simulink library "atmosphere2"  (R2024b)
settings: Solver=VariableStepAuto  StartTime=0.0  StopTime=10.0  RelTol=1e-3
libraries: $bdroot x14
settings Model: Creator=user  LastModifiedBy=user

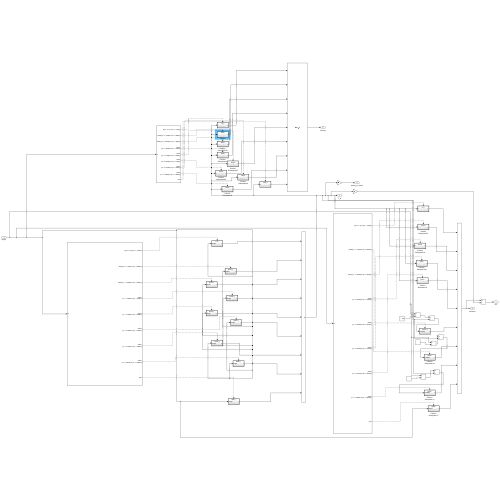
[thumbnail: Simulink's stored preview of the top-level diagram]
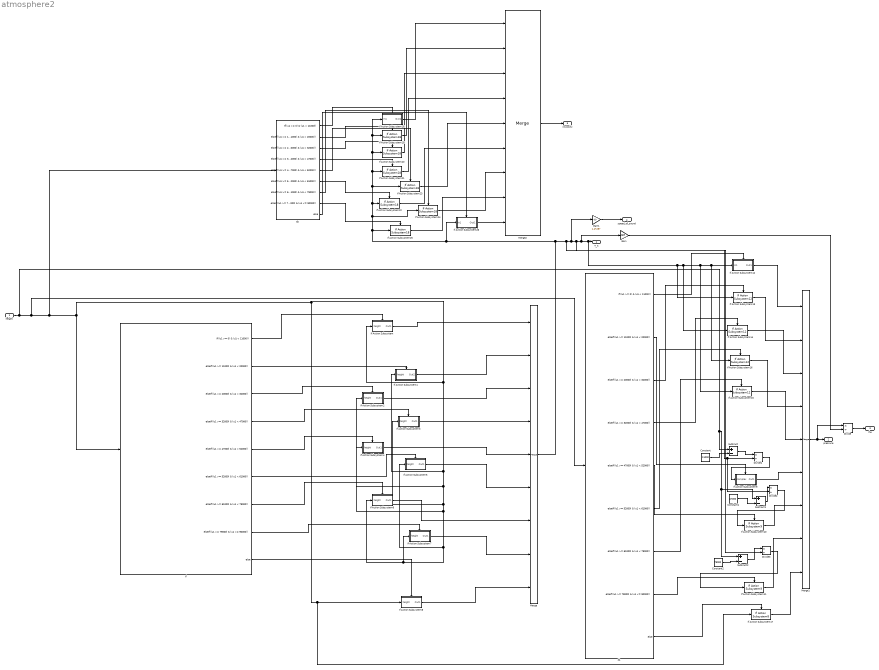
== system atmosphere2 ==
  height : Inport
  Constant : Constant  Value=11000
  Constant1 : Constant  Value=47000
  Constant2 : Constant  Value=79000
  Divide{,1..3} (4 alike) : Product  Inputs=*/
  Gain : Gain  Gain=287
  Gain1 : Gain  Gain=1.4*287
  If : If  IfExpression=(u1 >= 0) & (u1 < 11000)  ElseIfExpressions=|
      | (u1 >= 11000) & (u1 < 20000), (u1 >= 20000) & (u1 < 32000),
      | (u1 >= 32000) & (u1 < 47000),
      | (u1 >= 47000) & (u1 < 52000),
      | (u1 >= 52000) & (u1 < 61000),
      | (u1 >= 61000) & (u1 < 79000),
      | (u1 >= 79000) & (u1 <= 90000)
  If Action Subsystem : Subsystem  TreatAsAtomicUnit=on
  If Action Subsystem1 : Subsystem  TreatAsAtomicUnit=on
  If Action Subsystem10 : $bdroot/If Action Subsystem9  SystemSampleTime=-1  VariantActivationTime=update diagram  AllowFlexibleInterface=on  Latency=0  AutoFrameSizeCalculation=off
      link override Constant: Value=47000
      link override Gain: Gain=110.91
  If Action Subsystem11 : $bdroot/If Action Subsystem9  SystemSampleTime=-1  VariantActivationTime=update diagram  AllowFlexibleInterface=on  Latency=0  AutoFrameSizeCalculation=off
      link override Gain: Gain=0.373
  If Action Subsystem12 : Subsystem  TreatAsAtomicUnit=on
  If Action Subsystem13 : $bdroot/If Action Subsystem12  SystemSampleTime=-1  VariantActivationTime=update diagram  AllowFlexibleInterface=on  Latency=0  AutoFrameSizeCalculation=off
      link override Constant: Value=216.65
      link override g//8r*K): Value=-9.80665/(0.001*287)
  If Action Subsystem14 : $bdroot/If Action Subsystem12  SystemSampleTime=-1  VariantActivationTime=update diagram  AllowFlexibleInterface=on  Latency=0  AutoFrameSizeCalculation=off
      link override Constant: Value=228.65
      link override Gain: Gain=868.02
      link override g//8r*K): Value=-9.80665/(-0.0028*287)
  If Action Subsystem15 : $bdroot/If Action Subsystem12  SystemSampleTime=-1  VariantActivationTime=update diagram  AllowFlexibleInterface=on  Latency=0  AutoFrameSizeCalculation=off
      link override Constant: Value=252.65
      link override Gain: Gain=1.82
      link override g//8r*K): Value=-9.80665/(-0.004*287)
  If Action Subsystem16 : $bdroot/If Action Subsystem12  SystemSampleTime=-1  VariantActivationTime=update diagram  AllowFlexibleInterface=on  Latency=0  AutoFrameSizeCalculation=off
      link override Constant: Value=270.65
      link override Gain: Gain=59
      link override g//8r*K): Value=-9.80665/(-0.002*287)
  If Action Subsystem17 : $bdroot/If Action Subsystem8  SystemSampleTime=-1  VariantActivationTime=update diagram  AllowFlexibleInterface=on  Latency=0  AutoFrameSizeCalculation=off
  If Action Subsystem18 : Subsystem  TreatAsAtomicUnit=on
  If Action Subsystem19 : $bdroot/If Action Subsystem18  SystemSampleTime=-1  VariantActivationTime=update diagram  AllowFlexibleInterface=on  Latency=0  AutoFrameSizeCalculation=off
      link override Constant: Value=216.65
      link override Constant2: Value=216.65
  If Action Subsystem2 : Subsystem  TreatAsAtomicUnit=on
  If Action Subsystem20 : $bdroot/If Action Subsystem18  SystemSampleTime=-1  VariantActivationTime=update diagram  AllowFlexibleInterface=on  Latency=0  AutoFrameSizeCalculation=off
      link override Constant: Value=216.65
      link override Constant2: Value=216.65
  If Action Subsystem21 : $bdroot/If Action Subsystem18  SystemSampleTime=-1  VariantActivationTime=update diagram  AllowFlexibleInterface=on  Latency=0  AutoFrameSizeCalculation=off
      link override Constant: Value=228.65
      link override Constant2: Value=228.65
  If Action Subsystem22 : $bdroot/If Action Subsystem18  SystemSampleTime=-1  VariantActivationTime=update diagram  AllowFlexibleInterface=on  Latency=0  AutoFrameSizeCalculation=off
      link override Constant: Value=270.65
      link override Constant2: Value=270.65
  If Action Subsystem23 : $bdroot/If Action Subsystem18  SystemSampleTime=-1  VariantActivationTime=update diagram  AllowFlexibleInterface=on  Latency=0  AutoFrameSizeCalculation=off
      link override Constant: Value=270.65
      link override Constant2: Value=270.65
  If Action Subsystem24 : $bdroot/If Action Subsystem18  SystemSampleTime=-1  VariantActivationTime=update diagram  AllowFlexibleInterface=on  Latency=0  AutoFrameSizeCalculation=off
      link override Constant: Value=180.65
      link override Constant2: Value=180.65
  If Action Subsystem25 : $bdroot/If Action Subsystem18  SystemSampleTime=-1  VariantActivationTime=update diagram  AllowFlexibleInterface=on  Latency=0  AutoFrameSizeCalculation=off
      link override Constant: Value=180.65
      link override Constant2: Value=180.65
  If Action Subsystem26 : Subsystem  TreatAsAtomicUnit=on
  If Action Subsystem3 : Subsystem  TreatAsAtomicUnit=on
  If Action Subsystem4 : Subsystem  TreatAsAtomicUnit=on
  If Action Subsystem5 : Subsystem  TreatAsAtomicUnit=on
  If Action Subsystem6 : Subsystem  TreatAsAtomicUnit=on
  If Action Subsystem7 : Subsystem  TreatAsAtomicUnit=on
  If Action Subsystem8 : Subsystem  TreatAsAtomicUnit=on
  If Action Subsystem9 : Subsystem  TreatAsAtomicUnit=on
  If1 : If  IfExpression=(u1 >= 0) & (u1 < 11000)  ElseIfExpressions=|
      | (u1 >= 11000) & (u1 < 20000), (u1 >= 20000) & (u1 < 32000),
      | (u1 >= 32000) & (u1 < 47000),
      | (u1 >= 47000) & (u1 < 52000),
      | (u1 >= 52000) & (u1 < 61000),
      | (u1 >= 61000) & (u1 < 79000),
      | (u1 >= 79000) & (u1 <= 90000)
  If2 : If  IfExpression=(u1 >= 0) & (u1 < 11000)  ElseIfExpressions=|
      | (u1 >= 11000) & (u1 < 20000), (u1 >= 20000) & (u1 < 32000),
      | (u1 >= 32000) & (u1 < 47000),
      | (u1 >= 47000) & (u1 < 52000),
      | (u1 >= 52000) & (u1 < 61000),
      | (u1 >= 61000) & (u1 < 79000),
      | (u1 >= 79000) & (u1 <= 90000)
  Merge : Merge  Inputs=9
  Merge1 : Merge  Inputs=9
  Merge2 : Merge  Inputs=9
  Subtract : Sum  Inputs=+-
  Subtract1 : Sum  Inputs=+-
  Subtract2 : Sum  Inputs=+-
  T_K : Outport
  pressure : Outport  Port=2
  rho : Outport  Port=3
  spead_of_sound : Outport  Port=4
  viscosity : Outport  Port=5
  wires:
  If/1 -> If Action Subsystem/Action
  If/2 -> If Action Subsystem1/Action
  If/3 -> If Action Subsystem2/Action
  If/4 -> If Action Subsystem3/Action
  If/5 -> If Action Subsystem4/Action
  If/6 -> If Action Subsystem5/Action
  If/7 -> If Action Subsystem6/Action
  If/8 -> If Action Subsystem7/Action
  If/9 -> If Action Subsystem8/Action
  height/1 -> Subtract2/1, Subtract1/1, Subtract/1, If1/1, If2/1, If Action Subsystem4/1("height "), If Action Subsystem7/1("height "), If Action Subsystem6/1("height "), If Action Subsystem5/1("height "), If Action Subsystem3/1("height "), If Action Subsystem2/1("height "), If Action Subsystem1/1("height "), If Action Subsystem/1("height "), If Action Subsystem17/1, If Action Subsystem8/1("height "), If/1
  Merge/1 -> Divide3/2, Gain1/1, Divide2/2, Divide1/2, Gain/1, If Action Subsystem13/1, If Action Subsystem14/1, If Action Subsystem15/1, If Action Subsystem16/1, If Action Subsystem12/1(In1), T_K/1, If Action Subsystem24/1, If Action Subsystem22/1, If Action Subsystem23/1, If Action Subsystem21/1, If Action Subsystem20/1, If Action Subsystem19/1, If Action Subsystem18/1(In1), If Action Subsystem25/1, If Action Subsystem26/1(In1)
  If Action Subsystem/1(Out1) -> Merge/1
  If Action Subsystem1/1(Out2) -> Merge/2
  If Action Subsystem2/1(Out1) -> Merge/3
  If Action Subsystem3/1(Out1) -> Merge/4
  If Action Subsystem4/1(Out1) -> Merge/5
  If Action Subsystem5/1(Out1) -> Merge/6
  If Action Subsystem6/1(Out1) -> Merge/7
  If Action Subsystem7/1(Out1) -> Merge/8
  If Action Subsystem8/1(Out1) -> Merge/9
  If1/1 -> If Action Subsystem12/Action
  If1/3 -> If Action Subsystem13/Action
  If1/4 -> If Action Subsystem14/Action
  If1/6 -> If Action Subsystem16/Action
  If1/7 -> If Action Subsystem15/Action
  Constant/1 -> Subtract/2
  Subtract/1 -> Divide1/1
  Divide1/1 -> If Action Subsystem9/1(complex)
  If1/2 -> If Action Subsystem9/Action
  If1/5 -> If Action Subsystem10/Action
  Constant1/1 -> Subtract1/2
  Subtract1/1 -> Divide2/1
  Divide2/1 -> If Action Subsystem10/1
  If1/8 -> If Action Subsystem11/Action
  Constant2/1 -> Subtract2/2
  Subtract2/1 -> Divide3/1
  Divide3/1 -> If Action Subsystem11/1
  If Action Subsystem12/1(Out1) -> Merge1/1
  If Action Subsystem13/1 -> Merge1/2
  If Action Subsystem14/1 -> Merge1/3
  If Action Subsystem16/1 -> Merge1/4
  If Action Subsystem15/1 -> Merge1/5
  If Action Subsystem9/1(Out1) -> Merge1/6
  If Action Subsystem10/1 -> Merge1/7
  If Action Subsystem11/1 -> Merge1/8
  If Action Subsystem17/1 -> Merge1/9
  Merge1/1 -> Divide/1, pressure/1
  If1/9 -> If Action Subsystem17/Action
  Divide/1 -> rho/1
  Gain1/1 -> spead_of_sound/1
  If2/1 -> If Action Subsystem18/Action
  If2/2 -> If Action Subsystem19/Action
  If2/3 -> If Action Subsystem20/Action
  If2/4 -> If Action Subsystem21/Action
  If2/5 -> If Action Subsystem23/Action
  If2/6 -> If Action Subsystem22/Action
  If2/7 -> If Action Subsystem24/Action
  If2/8 -> If Action Subsystem25/Action
  If2/9 -> If Action Subsystem26/Action
  If Action Subsystem18/1(Out1) -> Merge2/1
  If Action Subsystem19/1 -> Merge2/2
  If Action Subsystem20/1 -> Merge2/3
  If Action Subsystem21/1 -> Merge2/4
  If Action Subsystem23/1 -> Merge2/5
  If Action Subsystem22/1 -> Merge2/6
  If Action Subsystem24/1 -> Merge2/7
  If Action Subsystem25/1 -> Merge2/8
  If Action Subsystem26/1(Out1) -> Merge2/9
  Merge2/1 -> viscosity/1
  Gain/1 -> Divide/2

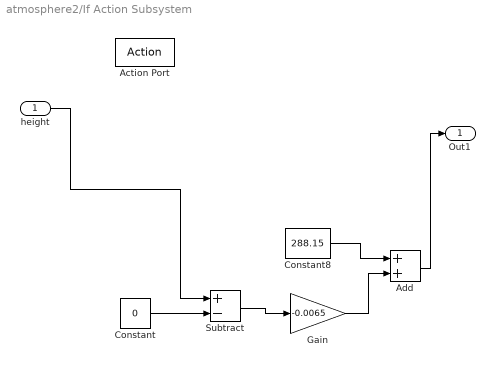
== system atmosphere2/If Action Subsystem ==
  "height " : Inport
  Action Port : ActionPort  ActionPortLabel=if((u1 >= 0) & (u1 < 11000))
  Add : Sum
  Constant : Constant  Value=0
  Constant8 : Constant  Value=288.15
  Gain : Gain  Gain=-0.0065
  Subtract : Sum  Inputs=+-
  Out1 : Outport
  wires:
  "height "/1 -> Subtract/1
  Constant/1 -> Subtract/2
  Subtract/1 -> Gain/1
  Gain/1 -> Add/2
  Constant8/1 -> Add/1
  Add/1 -> Out1/1

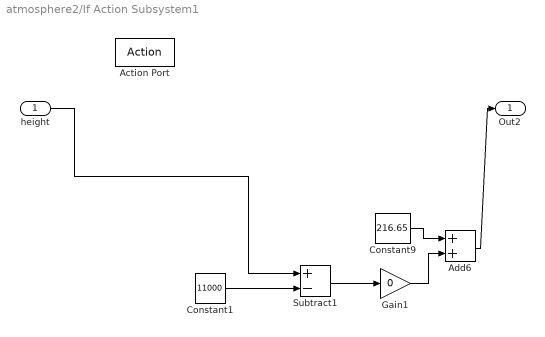
== system atmosphere2/If Action Subsystem1 ==
  "height " : Inport
  Action Port : ActionPort  ActionPortLabel=elseif((u1 >= 11000) & (u1 < 20000))
  Add6 : Sum
  Constant1 : Constant  Value=11000
  Constant9 : Constant  Value=216.65
  Gain1 : Gain  Gain=0
  Subtract1 : Sum  Inputs=+-
  Out2 : Outport
  wires:
  "height "/1 -> Subtract1/1
  Gain1/1 -> Add6/2
  Constant9/1 -> Add6/1
  Subtract1/1 -> Gain1/1
  Constant1/1 -> Subtract1/2
  Add6/1 -> Out2/1

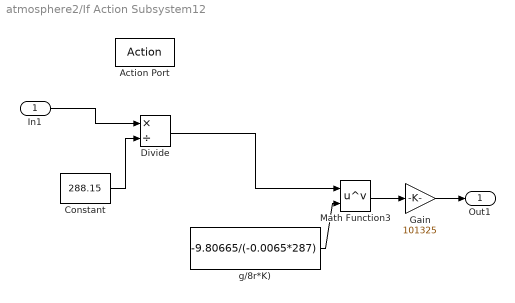
== system atmosphere2/If Action Subsystem12 ==
  In1 : Inport
  Action Port : ActionPort  ActionPortLabel=if((u1 >= 0) & (u1 < 11000))
  Constant : Constant  Value=288.15
  Divide : Product  Inputs=*/
  Gain : Gain  Gain=101325
  Math Function3 : Math  Operator=pow
  g/8r*K) : Constant  Value=-9.80665/(-0.0065*287)
  Out1 : Outport
  wires:
  In1/1 -> Divide/1
  Constant/1 -> Divide/2
  g/8r*K)/1 -> Math Function3/2
  Divide/1 -> Math Function3/1
  Math Function3/1 -> Gain/1
  Gain/1 -> Out1/1

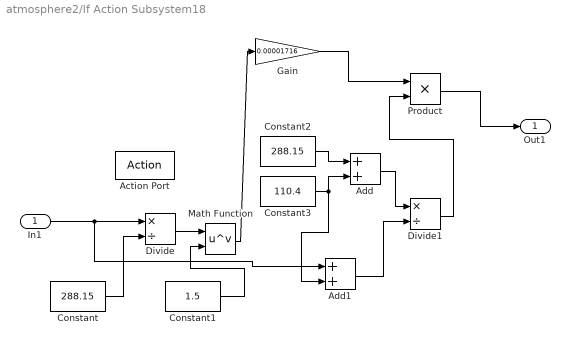
== system atmosphere2/If Action Subsystem18 ==
  In1 : Inport
  Action Port : ActionPort  ActionPortLabel=if((u1 >= 0) & (u1 < 11000))
  Add : Sum
  Add1 : Sum
  Constant : Constant  Value=288.15
  Constant1 : Constant  Value=1.5
  Constant2 : Constant  Value=288.15
  Constant3 : Constant  Value=110.4
  Divide : Product  Inputs=*/
  Divide1 : Product  Inputs=*/
  Gain : Gain  Gain=0.00001716
  Math Function : Math  Operator=pow
  Product : Product
  Out1 : Outport
  wires:
  In1/1 -> Add1/1, Divide/1
  Constant/1 -> Divide/2
  Divide/1 -> Math Function/1
  Constant1/1 -> Math Function/2
  Constant2/1 -> Add/1
  Constant3/1 -> Add/2, Add1/2
  Add/1 -> Divide1/1
  Add1/1 -> Divide1/2
  Divide1/1 -> Product/2
  Math Function/1 -> Gain/1
  Gain/1 -> Product/1
  Product/1 -> Out1/1

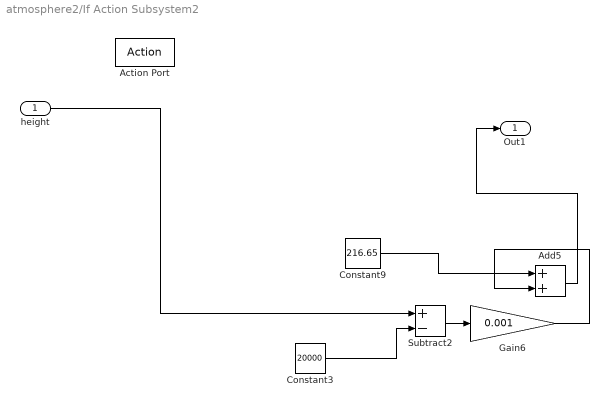
== system atmosphere2/If Action Subsystem2 ==
  "height " : Inport
  Action Port : ActionPort  ActionPortLabel=elseif( (u1 >= 20000) & (u1 < 32000))
  Add5 : Sum
  Constant3 : Constant  Value=20000
  Constant9 : Constant  Value=216.65
  Gain6 : Gain  Gain=0.001
  Subtract2 : Sum  Inputs=+-
  Out1 : Outport
  wires:
  Constant3/1 -> Subtract2/2
  Subtract2/1 -> Gain6/1
  Gain6/1 -> Add5/2
  Constant9/1 -> Add5/1
  "height "/1 -> Subtract2/1
  Add5/1 -> Out1/1

== system atmosphere2/If Action Subsystem26 ==
  In1 : Inport
  Action Port : ActionPort  ActionPortLabel=else
  Gain : Gain  Gain=0
  Out1 : Outport
  wires:
  In1/1 -> Gain/1
  Gain/1 -> Out1/1

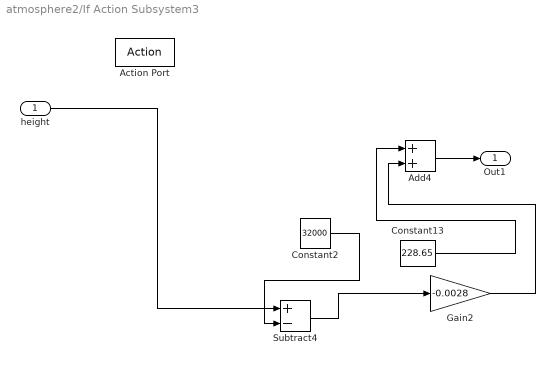
== system atmosphere2/If Action Subsystem3 ==
  "height " : Inport
  Action Port : ActionPort  ActionPortLabel=|
      | elseif(
      | (u1 >= 32000) & (u1 < 47000))
  Add4 : Sum
  Constant13 : Constant  Value=228.65
  Constant2 : Constant  Value=32000
  Gain2 : Gain  Gain=-0.0028
  Subtract4 : Sum  Inputs=+-
  Out1 : Outport
  wires:
  Subtract4/1 -> Gain2/1
  Constant2/1 -> Subtract4/2
  Constant13/1 -> Add4/1
  Gain2/1 -> Add4/2
  "height "/1 -> Subtract4/1
  Add4/1 -> Out1/1

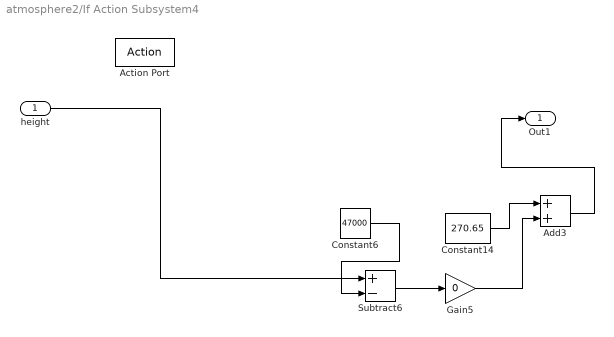
== system atmosphere2/If Action Subsystem4 ==
  "height " : Inport
  Action Port : ActionPort  ActionPortLabel=|
      | elseif(
      | (u1 >= 47000) & (u1 < 52000))
  Add3 : Sum
  Constant14 : Constant  Value=270.65
  Constant6 : Constant  Value=47000
  Gain5 : Gain  Gain=0
  Subtract6 : Sum  Inputs=+-
  Out1 : Outport
  wires:
  Subtract6/1 -> Gain5/1
  Constant14/1 -> Add3/1
  Constant6/1 -> Subtract6/2
  Gain5/1 -> Add3/2
  "height "/1 -> Subtract6/1
  Add3/1 -> Out1/1

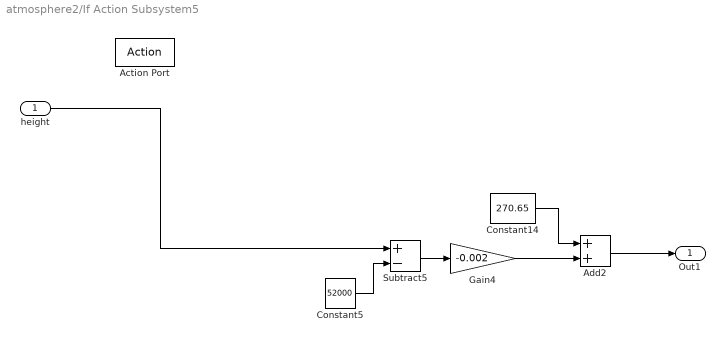
== system atmosphere2/If Action Subsystem5 ==
  "height " : Inport
  Action Port : ActionPort  ActionPortLabel=|
      | elseif(
      | (u1 >= 52000) & (u1 < 61000))
  Add2 : Sum
  Constant14 : Constant  Value=270.65
  Constant5 : Constant  Value=52000
  Gain4 : Gain  Gain=-0.002
  Subtract5 : Sum  Inputs=+-
  Out1 : Outport
  wires:
  Subtract5/1 -> Gain4/1
  Gain4/1 -> Add2/2
  Constant5/1 -> Subtract5/2
  Constant14/1 -> Add2/1
  "height "/1 -> Subtract5/1
  Add2/1 -> Out1/1

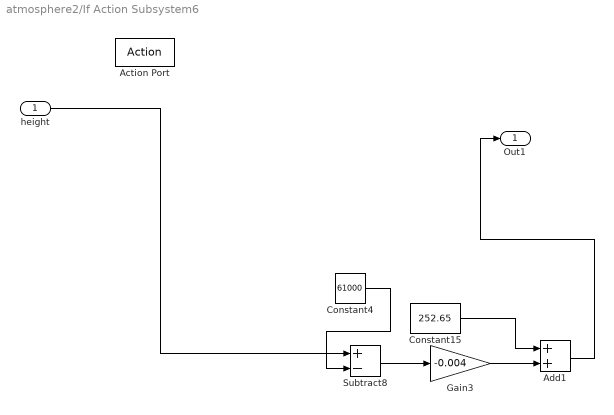
== system atmosphere2/If Action Subsystem6 ==
  "height " : Inport
  Action Port : ActionPort  ActionPortLabel=|
      | elseif(
      | (u1 >= 61000) & (u1 < 79000))
  Add1 : Sum
  Constant15 : Constant  Value=252.65
  Constant4 : Constant  Value=61000
  Gain3 : Gain  Gain=-0.004
  Subtract8 : Sum  Inputs=+-
  Out1 : Outport
  wires:
  Constant4/1 -> Subtract8/2
  Subtract8/1 -> Gain3/1
  Gain3/1 -> Add1/2
  Constant15/1 -> Add1/1
  "height "/1 -> Subtract8/1
  Add1/1 -> Out1/1

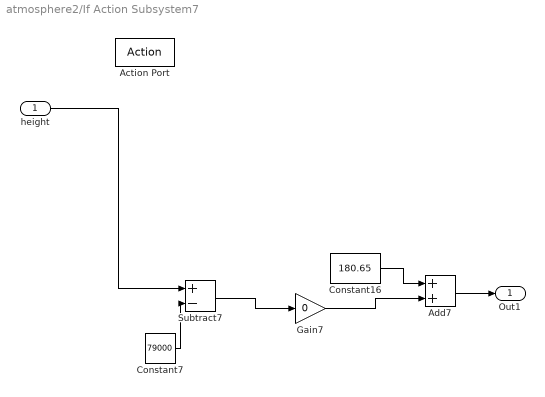
== system atmosphere2/If Action Subsystem7 ==
  "height " : Inport
  Action Port : ActionPort  ActionPortLabel=|
      | elseif(
      | (u1 >= 79000) & (u1 <= 90000))
  Add7 : Sum
  Constant16 : Constant  Value=180.65
  Constant7 : Constant  Value=79000
  Gain7 : Gain  Gain=0
  Subtract7 : Sum  Inputs=+-
  Out1 : Outport
  wires:
  Subtract7/1 -> Gain7/1
  Constant7/1 -> Subtract7/2
  Gain7/1 -> Add7/2
  Constant16/1 -> Add7/1
  "height "/1 -> Subtract7/1
  Add7/1 -> Out1/1

== system atmosphere2/If Action Subsystem8 ==
  "height " : Inport
  Action Port : ActionPort  ActionPortLabel=else
  Gain : Gain  Gain=0
  Out1 : Outport
  wires:
  "height "/1 -> Gain/1
  Gain/1 -> Out1/1

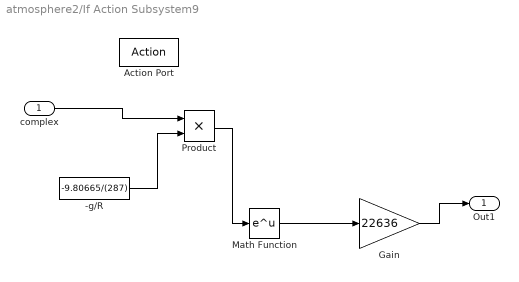
== system atmosphere2/If Action Subsystem9 ==
  complex : Inport
  Action Port : ActionPort  ActionPortLabel=elseif((u1 >= 11000) & (u1 < 20000))
  -g/R : Constant  Value=-9.80665/(287)
  Gain : Gain  Gain=22636
  Math Function : Math
  Product : Product
  Out1 : Outport
  wires:
  complex/1 -> Product/1
  -g/R/1 -> Product/2
  Math Function/1 -> Gain/1
  Product/1 -> Math Function/1
  Gain/1 -> Out1/1
